simulink model "PIDchr"  (R2020a)
settings: Solver=VariableStepAuto  StartTime=0.0  StopTime=20  RelTol=1e-5
settings Model: Creator=batis  LastModifiedBy=batis

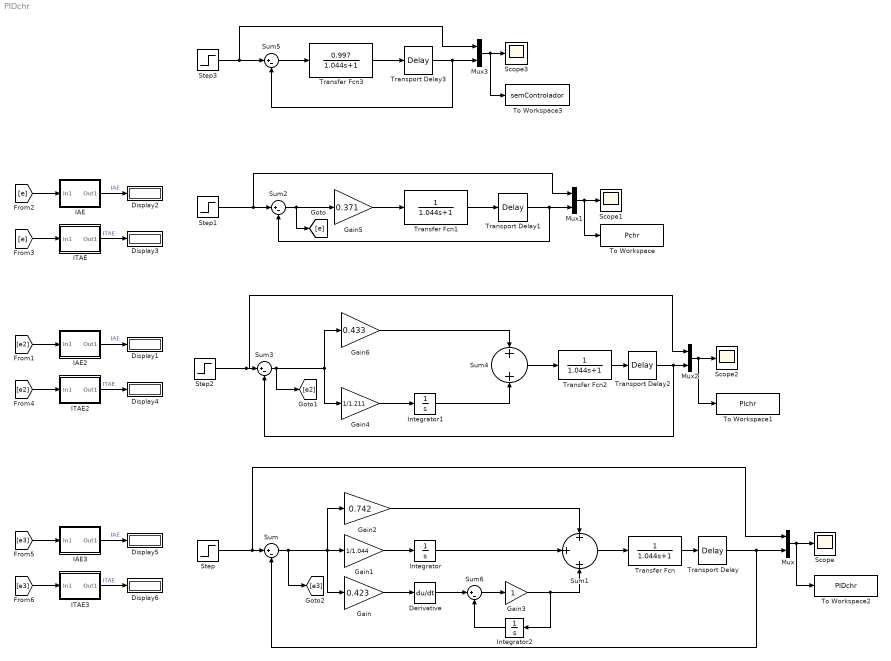
== system PIDchr ==
  Derivative : Derivative
  Display{1..6} (6 alike) : Display
  Gain : Gain  Gain=0.423
  Gain1 : Gain  Gain=1/1.044
  Gain2 : Gain  Gain=0.742
  Gain3 : Gain
  Gain4 : Gain  Gain=1/1.211
  Gain5 : Gain  Gain=0.371
  Gain6 : Gain  Gain=0.433
  IAE : Subsystem
  IAE2 : Subsystem
  IAE3 : Subsystem
  ITAE : Subsystem
  ITAE2 : Subsystem
  ITAE3 : Subsystem
  Integrator : Integrator
  Integrator1 : Integrator
  Integrator2 : Integrator
  Mux{,1..3} (4 alike) : Mux  Inputs=2
  Scope{,1..3} (4 alike) : Scope
  Step{,1..3} (4 alike) : Step  After=3  SampleTime=0
  Sum{,2..3,5..6} (5 alike) : Sum  Inputs=|+-
  Sum1 : Sum  Inputs=+|+|+
  Sum4 : Sum  Inputs=+|+
  To Workspace : ToWorkspace  VariableName=Pchr  SaveFormat=Structure With Time  SampleTime=-1
  To Workspace1 : ToWorkspace  VariableName=PIchr  SaveFormat=Structure With Time  SampleTime=-1
  To Workspace2 : ToWorkspace  VariableName=PIDchr  SaveFormat=Structure With Time  SampleTime=-1
  To Workspace3 : ToWorkspace  VariableName=semControlador  SaveFormat=Structure With Time  SampleTime=-1
  Transfer Fcn : TransferFcn  Denominator=[1.044 1]
  Transfer Fcn1 : TransferFcn  Denominator=[1.044 1]
  Transfer Fcn2 : TransferFcn  Denominator=[1.044 1]
  Transfer Fcn3 : TransferFcn  Numerator=[0.997]  Denominator=[1.044 1]
  Transport Delay : TransportDelay  DelayTime=0.846
  Transport Delay1 : TransportDelay  DelayTime=0.846  FixedBuffer=on
  Transport Delay2 : TransportDelay  DelayTime=0.846
  Transport Delay3 : TransportDelay  DelayTime=0.846  FixedBuffer=on
  wires:
  Sum/1 -> Gain/1, Gain2/1, Gain1/1, [e3]
  Sum1/1 -> Transfer Fcn/1
  Step/1 -> Sum/1, Mux/1
  Mux/1 -> To Workspace2/1, Scope/1
  Gain/1 -> Derivative/1
  Transfer Fcn/1 -> Transport Delay/1
  Transport Delay/1 -> Mux/2, Sum/2
  Gain2/1 -> Sum1/1
  Gain1/1 -> Integrator/1
  Integrator/1 -> Sum1/2
  Mux1/1 -> To Workspace/1, Scope1/1
  Sum2/1 -> [e], Gain5/1
  Gain5/1 -> Transfer Fcn1/1
  Step1/1 -> Sum2/1, Mux1/1
  Transfer Fcn1/1 -> Transport Delay1/1
  Transport Delay1/1 -> Mux1/2, Sum2/2
  Gain6/1 -> Sum4/1
  Transport Delay2/1 -> Mux2/2, Sum3/2
  Mux2/1 -> To Workspace1/1, Scope2/1
  Sum3/1 -> Gain6/1, Gain4/1, [e2]
  Gain4/1 -> Integrator1/1
  Transfer Fcn2/1 -> Transport Delay2/1
  Integrator1/1 -> Sum4/2
  Sum4/1 -> Transfer Fcn2/1
  Step2/1 -> Mux2/1, Sum3/1
  Transport Delay3/1 -> Mux3/2, Sum5/2
  Step3/1 -> Sum5/1, Mux3/1
  Transfer Fcn3/1 -> Transport Delay3/1
  Mux3/1 -> To Workspace3/1, Scope3/1
  Sum5/1 -> Transfer Fcn3/1
  Derivative/1 -> Sum6/1
  Sum6/1 -> Gain3/1
  Gain3/1 -> Integrator2/1, Sum1/3
  Integrator2/1 -> Sum6/2
  [e2] -> ITAE2/1(In1)
  IAE2/1(Out1) -> Display1/1  "IAE"
  [e2] -> IAE2/1(In1)
  ITAE2/1(Out1) -> Display4/1  "ITAE"
  [e] -> ITAE/1(In1)
  IAE/1(Out1) -> Display2/1  "IAE"
  ITAE/1(Out1) -> Display3/1  "ITAE"
  [e] -> IAE/1(In1)
  ITAE3/1(Out1) -> Display6/1  "ITAE"
  [e3] -> ITAE3/1(In1)
  IAE3/1(Out1) -> Display5/1  "IAE"
  [e3] -> IAE3/1(In1)

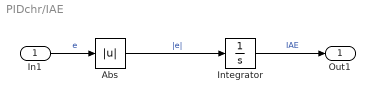
== system PIDchr/IAE ==
  In1 : Inport
  Abs : Abs
  Integrator : Integrator
  Out1 : Outport
  wires:
  Integrator/1 -> Out1/1  "IAE"
  In1/1 -> Abs/1  "e"
  Abs/1 -> Integrator/1  "|e|"

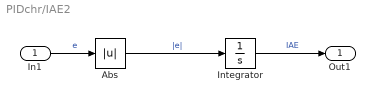
== system PIDchr/IAE2 ==
  In1 : Inport
  Abs : Abs
  Integrator : Integrator
  Out1 : Outport
  wires:
  Integrator/1 -> Out1/1  "IAE"
  In1/1 -> Abs/1  "e"
  Abs/1 -> Integrator/1  "|e|"

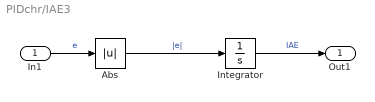
== system PIDchr/IAE3 ==
  In1 : Inport
  Abs : Abs
  Integrator : Integrator
  Out1 : Outport
  wires:
  Integrator/1 -> Out1/1  "IAE"
  In1/1 -> Abs/1  "e"
  Abs/1 -> Integrator/1  "|e|"

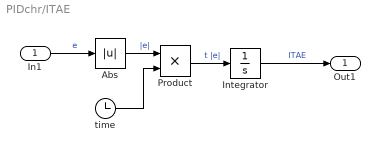
== system PIDchr/ITAE ==
  In1 : Inport
  Abs : Abs
  Integrator : Integrator
  Product : Product
  time : Clock
  Out1 : Outport
  wires:
  In1/1 -> Abs/1  "e"
  Integrator/1 -> Out1/1  "ITAE"
  time/1 -> Product/2
  Abs/1 -> Product/1  "|e|"
  Product/1 -> Integrator/1  "t |e|"

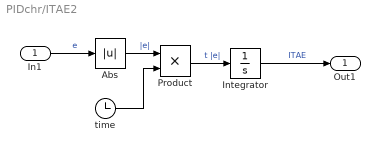
== system PIDchr/ITAE2 ==
  In1 : Inport
  Abs : Abs
  Integrator : Integrator
  Product : Product
  time : Clock
  Out1 : Outport
  wires:
  In1/1 -> Abs/1  "e"
  Integrator/1 -> Out1/1  "ITAE"
  time/1 -> Product/2
  Abs/1 -> Product/1  "|e|"
  Product/1 -> Integrator/1  "t |e|"

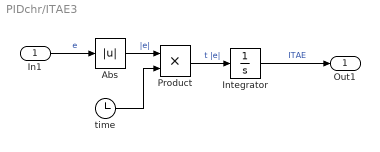
== system PIDchr/ITAE3 ==
  In1 : Inport
  Abs : Abs
  Integrator : Integrator
  Product : Product
  time : Clock
  Out1 : Outport
  wires:
  In1/1 -> Abs/1  "e"
  Integrator/1 -> Out1/1  "ITAE"
  time/1 -> Product/2
  Abs/1 -> Product/1  "|e|"
  Product/1 -> Integrator/1  "t |e|"
